simulink model "flight_model_1d"  (R2025b)
settings: Solver=VariableStepAuto  StartTime=0.0  StopTime=10.0  RelTol=1e-3
undefined symbols (not defined in the file): mass
settings Model: Creator=karadeli  LastModifiedBy=karadeli

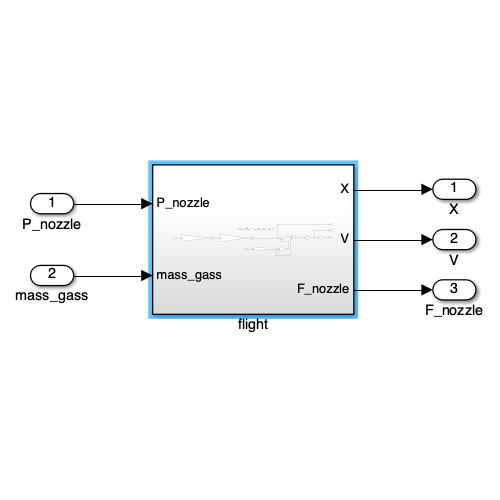
[thumbnail: Simulink's stored preview of the top-level diagram]
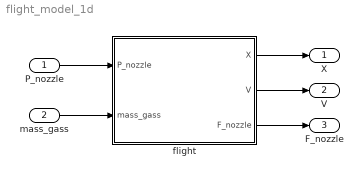
== system flight_model_1d ==
  P_nozzle : Inport  Unit=bar
  mass_gass : Inport  Port=2  Unit=bar
  flight : Subsystem
  X : Outport
  V : Outport  Port=2
  F_nozzle : Outport  Port=3
  wires:
  P_nozzle/1 -> flight/1(P_nozzle)
  mass_gass/1 -> flight/2(mass_gass)
  flight/1(X) -> X/1
  flight/2(V) -> V/1
  flight/3(F_nozzle) -> F_nozzle/1

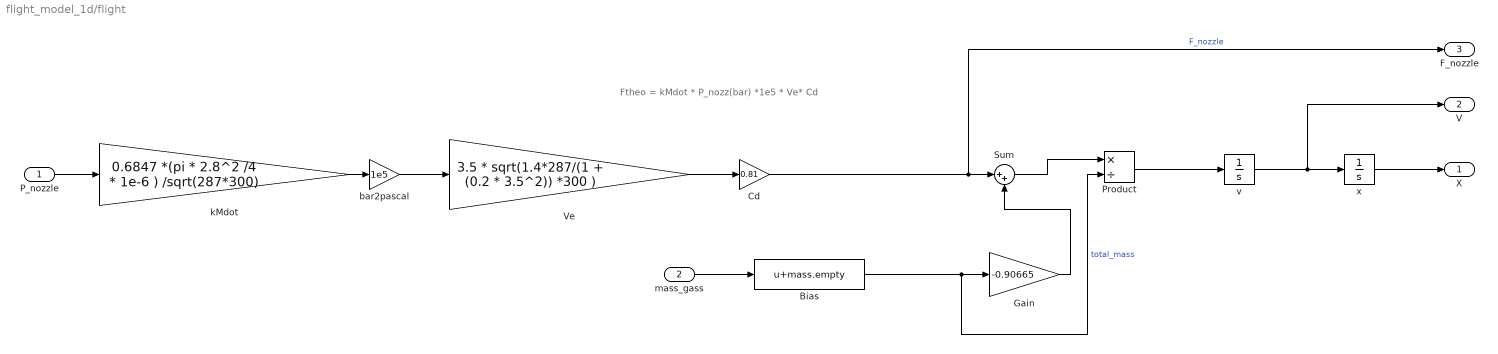
== system flight_model_1d/flight ==
  note: Ftheo = kMdot * P_nozz(bar) *1e5 * Ve* Cd
  P_nozzle : Inport  Unit=bar
  mass_gass : Inport  Port=2  Unit=bar
  Bias : Bias  Bias=mass.empty  SaturateOnIntegerOverflow=off
  Cd : Gain  Gain=0.81
  Gain : Gain  Gain=-0.90665
  Product : Product  Inputs=*/
  Sum : Sum  Inputs=|++
  Ve : Gain  Gain=3.5 * sqrt(1.4*287/(1 + (0.2 * 3.5^2)) *300 )
  bar2pascal : Gain  Gain=1e5
  kMdot : Gain  Gain=0.6847 *(pi * 2.8^2 /4 * 1e-6 ) /sqrt(287*300)
  v : Integrator
  x : Integrator  InitialCondition=9
  X : Outport
  V : Outport  Port=2
  F_nozzle : Outport  Port=3
  wires:
  Gain/1 -> Sum/2
  Sum/1 -> Product/1
  x/1 -> X/1
  kMdot/1 -> bar2pascal/1
  Bias/1 -> Product/2, Gain/1  "total_mass"
  bar2pascal/1 -> Ve/1
  Cd/1 -> F_nozzle/1, Sum/1  "F_nozzle"
  Product/1 -> v/1
  Ve/1 -> Cd/1
  P_nozzle/1 -> kMdot/1
  mass_gass/1 -> Bias/1
  v/1 -> V/1, x/1
